simulink model "PerformanceAnalysis"  (R2020a)
settings: Solver=FixedStepDiscrete  StartTime=0.0  StopTime=T  FixedStep=Ts  RelTol=1e-3
PreLoadFcn:
  | % Load all configuration
  | config;
values from neighbouring files (symbols this model uses):
  temp = 25    [config.m]
  Ts = 5e-6    (= 5e-06)    [GridConnectedDesignConfiguration.m]    (also in config.m = 1e-05)
undefined symbols (not defined in the file or in its folder): sigbuilder_block
libraries: powerlib x2, re_lib x1
settings Model: Creator=debma  LastModifiedBy=debma

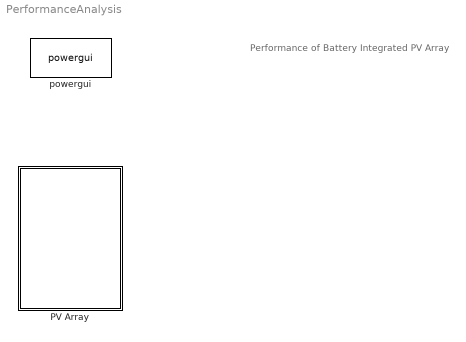
== system PerformanceAnalysis ==
  note: Performance of Battery Integrated PV Array
  PV Array : Subsystem
  powergui : powerlib/powergui  Priority=1  SimulationMode=Discrete  SampleTime=Ts  frequency=60  Iterations=50  frequencyindice=60  Pbase=100e6  ErrMax=1e-4  UnitsV=kV  UnitsW=MW  buscounter=0  FunctionMessages=off  echomessages=off  EnableUseOfTLC=off  CurrentSourceSwitches=off  DisableSnubberDevices=off  DisableRonSwitches=off  DisableVfSwitches=off  DisplayEquations=off  AutomaticDiscreteSolvers=off  SolverType=Tustin/Backward Euler (TBE)  Interpol=off  ExternalGateDelay=off  methode=off  Ts=100  x0status=blocks  SPID=on  SwTol=0  HookPort=off  NonlinearTolerance=1e-4  nMaxIteration=100  ContinueOnMaxIteration=off  RestoreLinks=warning  ResistiveCurrentMeasurement=off  Frange=[0:2:500]  Ylog=off  Xlog=on  ShowGrid=off  save=off  variable=ZData  structure=0  ZoomFFT=off  StartTime=0.0  cycles=1  DisplayStyle=1  fundamental=60  FreqAxis=off  MaxFrequency=1000  frequencyindicesteady=1  RmsSteady=1  display=off

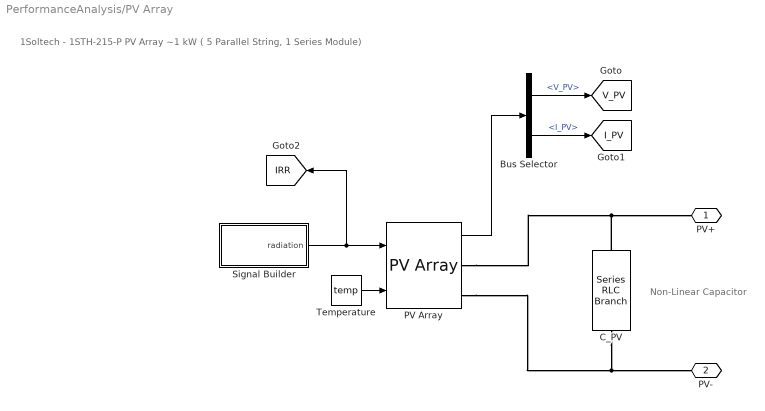
== system PerformanceAnalysis/PV Array ==
  note: 1Soltech - 1STH-215-P PV Array
      | ~1 kW ( 5 Parallel String, 1 Series Module)
  note: Non-Linear Capacitor
  Bus Selector : BusSelector  OutputSignals=V_PV,I_PV
  C_PV : powerlib/Elements/Series RLC Branch  LConnTagsString=__new0  RConnTagsString=__new0  BranchType=RLC  Resistance=1  Inductance=1e-3  SetiL0=off  InitialCurrent=0  Capacitance=1e-6  Setx0=off  InitialVoltage=0  Measurements=None
  PV Array : re_lib/Solar/PV Array  Npar=5  Nser=1  PlotType=array @ 1000 W/m2 & specified temperatures  S_vec="[ 1000  500  100 ]"  Temp_C_vec="[ 45 25  ]"  ModuleName=1Soltech 1STH-215-P  PlotWhenSelected=off  Pm=213.15  Ncell=60  Voc=36.3  Isc=7.84  Vm=29  Im=7.35  beta_Voc_pc=-0.36099  alpha_Isc_pc=0.102  beta_Voc=-0.13104  alpha_Isc=0.007997  IL=7.8649  I0=2.9259e-10  nI=0.98117  Rsh=313.3991  Rs=0.39383  RobustModel=off  RobustCellTemperature=25  BAL=on  Tc=1e-6  Tfilter=5e-5
  Signal Builder : Subsystem  Tag=STV Subsys  LoadFcn=sigbuilder_block('load');  StartFcn=sigbuilder_block('start');  StopFcn=sigbuilder_block('stop');  ClipboardFcn=sigbuilder_block('clipboard');  mask(Sigbuilder block){tuvar=[0:10]}
      mask help: Simulink:masks:SigbuilderBlock_MD
      mask init:
      | if ~strcmp(get_param(bdroot(gcbh),'SimulationStatus'),'stopped') tuvar = sigbuilder_block('maskInit'); end
      settings: CopyFcn=sigbuilder_block('copy');  DeleteFcn=sigbuilder_block('delete');  ModelCloseFcn=sigbuilder_block('modelClose');  PreSaveFcn=sigbuilder_block('preSave');  PauseFcn=sigbuilder_block('pause');  ContinueFcn=sigbuilder_block('continue');  NameChangeFcn=sigbuilder_block('namechange');  OpenFcn=sigbuilder_block('open',[0 30 1024.5 488.25 ]);  CloseFcn=sigbuilder_block('close');
      mask Display: plot(0, 0, 100, 100,[2, 2, 32, 32, 2], [68, 8, 8, 68, 68],[32, 2], [38, 38], [32, 19, 2],[53, 60, 44], [32, 17, 17, 2],[16, 16, 31, 31]);txt = getActiveGroup(gcbh);text(2, 100, txt,'verticalAlignment', 'top');
  Temperature : Constant  Value=temp
  PV+ : PMIOPort  Side=Right
  PV- : PMIOPort  Port=2  Side=Right
  tag scope: IRR=global, I_PV=global, V_PV=global
  wires:
  Temperature/1 -> PV Array/2
  Bus Selector/2 -> [I_PV]  "<I_PV>"
  PV Array/1 -> Bus Selector/1
  Bus Selector/1 -> [V_PV]  "<V_PV>"
  Signal Builder/1(radiation) -> [IRR], PV Array/1
  connections:
  PV Array/RConn1 -- PV+/RConn1 -- C_PV/LConn1
  PV Array/RConn2 -- C_PV/RConn1 -- PV-/RConn1

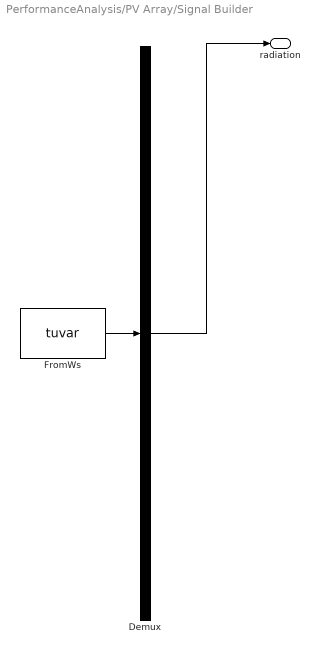
== system PerformanceAnalysis/PV Array/Signal Builder ==
  Demux : Demux  Tag=STV Demux  Outputs=1
      settings: DisplayOption=none
  FromWs : FromWorkspace  Tag=STV FromWs  VariableName=tuvar
      SigBuilderData=|
      | common.afterFinalStr = 'Extrapolate'
      | common.sampleTime = 0
      | dataSet.timeRange = [0 10]
      | dataSet.name = 'Group 1'
      | sbobj.Groups.Name = 'Group 1'
      | sbobj.Groups.Signals.Name = 'radiation'
      | sbobj.Groups.Signals.XData = [0 0.05 0.1 0.15 0.2 0.25 0.3 0.35 0.4 0.45 0.5 0.55 0.6 0.65 0.7 0.75 0.8 0.85 0.9 0.95 1 1.05 1.1 1.15 1.2 1.25 1.3 1.35 1.4 1.45 1.5 1.55 1.6 1.65 1.7 1.75 1.8 1.85 1.9 1.95 2 2.05 2.1 2.15 2.2 2.25 2.3 2.35 2.4 2.45 2.5 2.55 2.6 2.65 2.7 2.75 2.8 2.85 2.9 2.95 3 3.05 3.1 3.15 3.2 3.25 3.3 3.35 3.4 3.45 3.5 3.55 3.6 3.65 3.7 3.75 3.8 3.85 3.9 3.95 4 4.05 4.1 4.15 4.2 4.25 4.3 4.35 4.4 4.45 4.5 4.55 4.6 4.65 4.7 4.75 4.8 4.85 4.9 4.95 5 5.05 5.1 5.15 5.2 5.25 5.3 5.35 5.4 5.45 5.5 5.55 5.6 5.65 5.7 5.75 5.8 5.85 5.9 5.95 6 6.05 6.1 6.15 6.2 6.25 6.3 6.35 6.4 6.45 6.5 6.55 6.6 6.65 6.7 6.75 6.8 6.85 6.9 6.95 7 7.05 7.1 7.15 7.2 7.25 7.3 7.35 7.4 7.45 7.5 7.55 7.6 7.65 7.7 7.75 7.8 7.85 7.9 7.95 8 8.05 8.1 8.15 8.2 8.25 8.3 8.35 8.4 8.45 8.5 8.55 8.6 8.65 8.7 8.75 8.8 8.85 8.9 8.95 9 9.05 9.1 9.15 9.2 9.25 9.3 9.35 9.4 9.45 9.5 9.55 9.6 9.65 9.7 9.75 9.8 9.85 9.9 10]
      | sbobj.Groups.Signals.YData = [0 0 0 0 0 0 0 0 0 0 0 0 0 0 0 0 0 0 0 0 0 0 0 0 0 0 0 0 0 0 0 0 0 0 0 0 0 0 0 0 0 8.22e-08 0.003228513 0.034126005 0.096313816 0.172558216 0.250637465 0.324795877 0.392875749 0.45441224 0.509671489 0.559198015 0.603608707 0.643503063 0.679427759 0.711866261 0.741239613 0.76791177 0.792196398 0.814363714 0.83464677 0.853246984 0.870338888 0.886074162 0.900585024 0.913987092 0.926381772 0.937858272 0.948495295 0.958362463 0.967521526 0.97602738 0.983928938 0.991269869 0.998089232 1.004422016 1.010299608 1.015750197 1.020799114 1.025469142 1.029780769 1.033752418 1.037400642 1.040740298 1.043784695 1.046545723 1.049033969 1.051258811 1.05322851 1.054950275 1.056430334 1.05767398 1.058685622 1.059468819 1.060026308 1.06036003 1.060471142 1.06036003 1.060026308 1.059468819 1.058685622 1.05767398 1.056430334 1.054950275 1.05322851 1.051258811 1.049033969 1.046545723 1.043784695 1.040740298 1.037400642 1.033752418 1.029780769 1.025469142 1.020799114 1.015750197 1.010299608 1.004422016 0.998089232 0.991269869 0.983928938 0.97602738 0.967521526 0.958362463 0.948495295 0.937858272 0.926381772 0.913987092 0.900585024 0.886074162 0.870338888 0.853246984 0.83464677 0.814363714 0.792196398 0.76791177 0.741239613 0.711866261 0.679427759 0.643503063 0.603608707 0.559198015 0.509671489 0.45441224 0.392875749 0.324795877 0.250637465 0.172558216 0.096313816 0.034126005 0.003228513 8.22e-08 0 0 0 0 0 0 0 0 0 0 0 0 0 0 0 0 0 0 0 0 0 0 0 0 0 0 0 0 0 0 0 0 0 0 0 0 0 0 0 0 0 0 0 0 0 0 0 0]
  radiation : Outport  Tag=STV Outport
  wires:
  FromWs/1 -> Demux/1
  Demux/1 -> radiation/1
